simulink model "A1V1"  (R2023b)
settings: Solver=FixedStepAuto  StartTime=0.0  StopTime=10.0  FixedStep=1e-3  RelTol=1e-3  EnableMultiTasking=on
undefined symbols (not defined in the file): D0, D1, D10, D11, D12, D13, D2, D3, D4, D5, D6, D7, D8, D9, PTA0, PTA1, PTA2, PTB23, PTB9, PTC16, PTC17, PTC2, PTC3, PTC4, PTD0, PTD1, PTD2, PTD3
libraries: frdmk64flib x14
settings Model: ExtModeTrigDuration=5  Creator=aless  LastModifiedBy=aless
settings OptimizationCC: EnhancedBackFolding=on  PassReuseOutputArgsAs=Individual arguments  ZeroExternalMemoryAtStartup=off  ZeroInternalMemoryAtStartup=off  MaxStackSize=64  OptimizeBlockOrder=speed  DifferentSizesBufferReuse=on  OptimizationCustomize=off  EfficientTunableParamExpr=on
settings DebuggingCC: ParameterTunabilityLossMsg=error
settings HardwareCC: ProdBitPerPointer=32  ProdBitPerSizeT=32  ProdBitPerPtrDiffT=32  ProdLargestAtomicInteger=Long  ProdLargestAtomicFloat=Double  ProdWordSize=32  ProdHWDeviceType=ARM Compatible->ARM Cortex
settings SFSimCC: MATLABDynamicMemAlloc=off
settings RTWCC: Description=Embedded Coder  SystemTargetFile=ert.tlc  HardwareBoard=NXP FRDM-K64F  TLCOptions="-aInlineSetEventsForThisBaseRateFcn=TLC_FALSE -aSuppressMultiTaskScheduler=TLC_FALSE  -aRateBasedStepFcn=0"  TemplateMakefile=ert_default_tmf  Toolchain=GNU Tools for ARM Embedded Processors
settings CodeAppCC: ForceParamTrailComments=on  IgnoreCustomStorageClasses=off  OperatorAnnotations=on  SimulinkDataObjDesc=on  SFDataObjDesc=on  InsertBlockDesc=on
settings ERTTargetCC: ExtModeTransport=4  ExtModeMexFile=sendToCommService

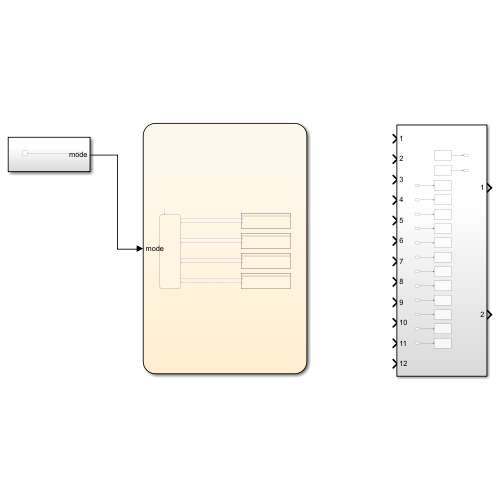
[thumbnail: Simulink's stored preview of the top-level diagram]
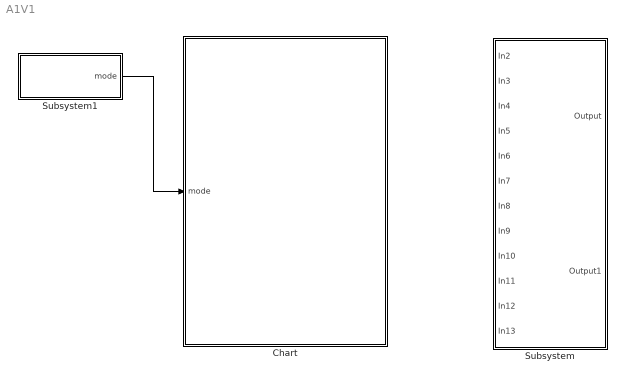
== system A1V1 ==
  Chart : Stateflow chart  TreatAsAtomicUnit=on
  Subsystem : Subsystem
  Subsystem1 : Subsystem
  wires:
  Subsystem1/1(mode) -> Chart/1(mode)

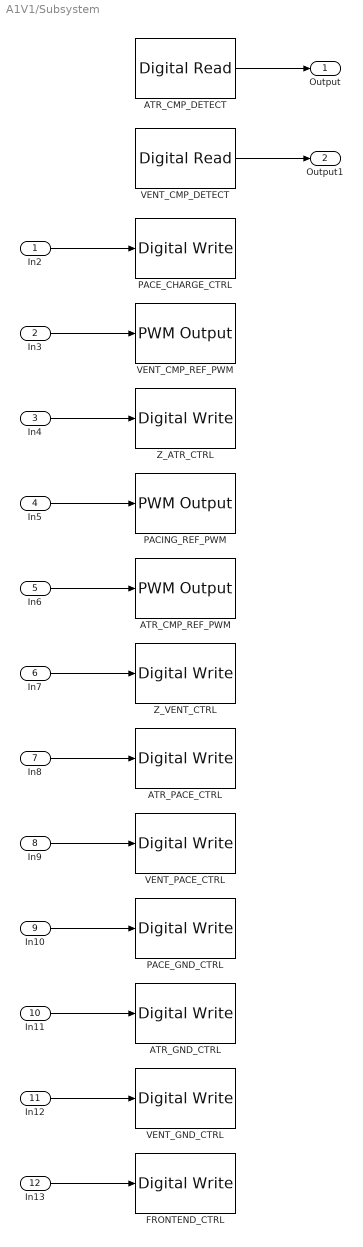
== system A1V1/Subsystem ==
  In2 : Inport
  In3 : Inport  Port=2
  In4 : Inport  Port=3
  In5 : Inport  Port=4
  In6 : Inport  Port=5
  In7 : Inport  Port=6
  In8 : Inport  Port=7
  In9 : Inport  Port=8
  In10 : Inport  Port=9
  In11 : Inport  Port=10
  In12 : Inport  Port=11
  In13 : Inport  Port=12
  ATR_CMP_DETECT : frdmk64flib/Digital Read  Whichpin=PTC16 (D0)  SampleTime=-1
  ATR_CMP_REF_PWM : frdmk64flib/PWM Output  Whichpin=PTC2 (D6)  InitialFrequency=2000  InitialDutyCycle=30
  ATR_GND_CTRL : frdmk64flib/Digital Write  Whichpin=PTD2 (D11)
  ATR_PACE_CTRL : frdmk64flib/Digital Write  Whichpin=PTA0 (D8)
  FRONTEND_CTRL : frdmk64flib/Digital Write  Whichpin=PTD1 (D13)
  PACE_CHARGE_CTRL : frdmk64flib/Digital Write  Whichpin=PTB9 (D2)
  PACE_GND_CTRL : frdmk64flib/Digital Write  Whichpin=PTD0 (D10)
  PACING_REF_PWM : frdmk64flib/PWM Output  Whichpin=PTA2 (D5)  InitialFrequency=2000  InitialDutyCycle=30
  VENT_CMP_DETECT : frdmk64flib/Digital Read  Whichpin=PTC17 (D1)  SampleTime=-1
  VENT_CMP_REF_PWM : frdmk64flib/PWM Output  Whichpin=PTA1 (D3)  InitialFrequency=2000  InitialDutyCycle=30
  VENT_GND_CTRL : frdmk64flib/Digital Write  Whichpin=PTD3 (D12)
  VENT_PACE_CTRL : frdmk64flib/Digital Write  Whichpin=PTC4 (D9)
  Z_ATR_CTRL : frdmk64flib/Digital Write  Whichpin=PTB23 (D4)
  Z_VENT_CTRL : frdmk64flib/Digital Write  Whichpin=PTC3 (D7)
  Output : Outport
  Output1 : Outport  Port=2
  wires:
  In11/1 -> ATR_GND_CTRL/1
  In5/1 -> PACING_REF_PWM/1
  In7/1 -> Z_VENT_CTRL/1
  In12/1 -> VENT_GND_CTRL/1
  In9/1 -> VENT_PACE_CTRL/1
  In6/1 -> ATR_CMP_REF_PWM/1
  In13/1 -> FRONTEND_CTRL/1
  In2/1 -> PACE_CHARGE_CTRL/1
  In8/1 -> ATR_PACE_CTRL/1
  In10/1 -> PACE_GND_CTRL/1
  VENT_CMP_DETECT/1 -> Output1/1
  ATR_CMP_DETECT/1 -> Output/1
  In4/1 -> Z_ATR_CTRL/1
  In3/1 -> VENT_CMP_REF_PWM/1

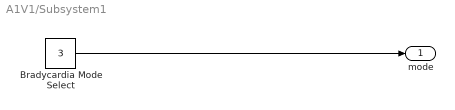
== system A1V1/Subsystem1 ==
  Bradycardia Mode Select : Constant  Value=3
  mode : Outport
  wires:
  Bradycardia Mode Select/1 -> mode/1

== stateflow chart A1V1/Chart ==
  state AOO [group]
    state Charging
    state Discharging
    AOO.Charging -> AOO.Discharging
    AOO.Discharging -> AOO.Charging
  state Mode
  state VOO [group]
    state Charging
    state Discharging
    VOO.Charging -> VOO.Discharging
    VOO.Discharging -> VOO.Charging
  state VVI [group]
    state Charging
    state Discharging
    VVI.Charging -> VVI.Discharging
    VVI.Discharging -> VVI.Charging
  state AAI [group]
    state Charging
    state Discharging
    AAI.Charging -> AAI.Discharging
    AAI.Discharging -> AAI.Charging
  (default) -> Mode [order 4] : [mode==1]
  (default) -> Mode [order 5] : [mode==0]
  (default) -> Mode [order 2] : [mode==2]
  (default) -> Mode [order 3] : [mode==1]
  Mode -> VVI.Charging [order 3] : [mode==2]
  Mode -> VOO.Charging [order 2] : [mode==1]
  Mode -> AOO.Charging [order 1] : [mode==0]
  (default) -> Mode [order 1]
  Mode -> AAI.Charging [order 4]
  data: mode input
